simulink model "vier_Bit_Subtractor"  (R2024b)
settings: Solver=VariableStepAuto  StartTime=0.0  StopTime=10.0  RelTol=1e-3
libraries: simulink x3
settings Model: Creator=Steve Kinfack  LastModifiedBy=Steve Kinfack

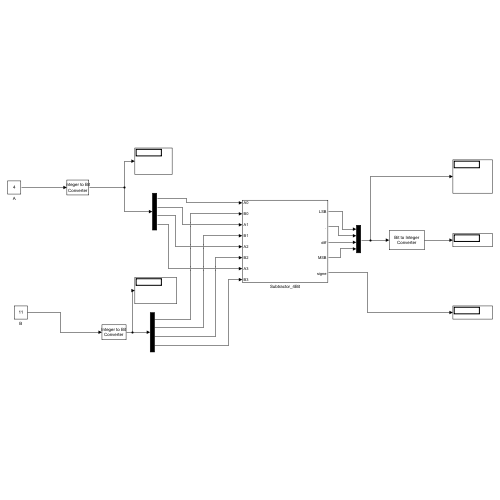
[thumbnail: Simulink's stored preview of the top-level diagram]
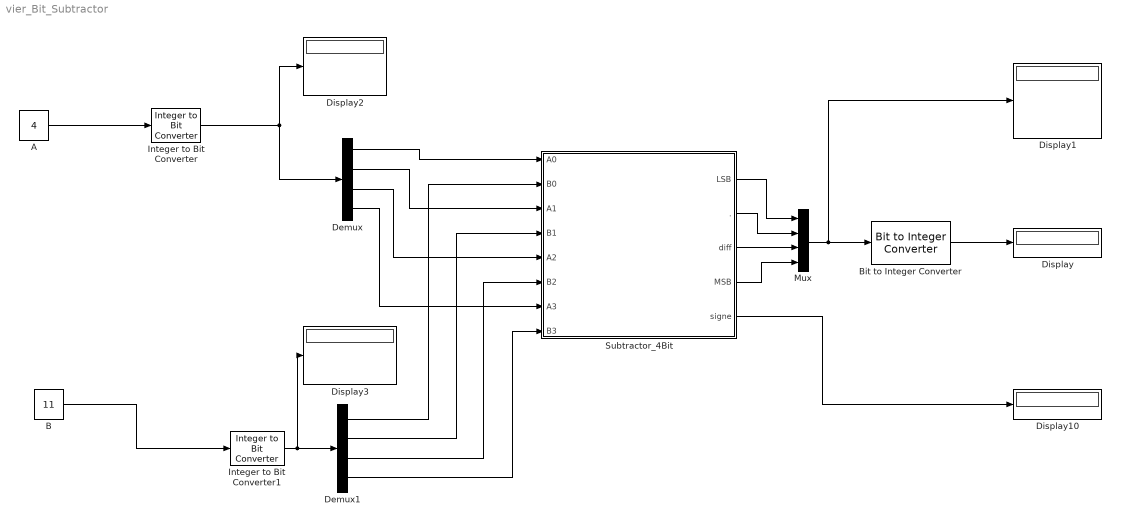
== system vier_Bit_Subtractor ==
  A : Constant  Value=4
  B : Constant  Value=11
  Bit to Integer Converter : simulink/Logic and Bit Operations/Bit to Integer Converter  nbits=4  bitOrder=LSB first  signedOutputValues=Unsigned  outDtype=Inherit via internal rule  outDtypeSigned=Inherit via internal rule
  Demux : Demux
  Demux1 : Demux
  Display{,1..3,10} (5 alike) : Display
  Integer to Bit Converter : simulink/Logic and Bit Operations/Integer to Bit Converter  nbits=4  signedInputValues=Unsigned  bitOrder=LSB first  outDtype=Inherit via internal rule
  Integer to Bit Converter1 : simulink/Logic and Bit Operations/Integer to Bit Converter  nbits=4  signedInputValues=Unsigned  bitOrder=LSB first  outDtype=Inherit via internal rule
  Mux : Mux
  Subtractor_4Bit : Subsystem
  wires:
  B/1 -> Integer to Bit Converter1/1
  Subtractor_4Bit/1(LSB) -> Mux/1
  Mux/1 -> Display1/1, Bit to Integer Converter/1
  Integer to Bit Converter/1 -> Demux/1, Display2/1
  Integer to Bit Converter1/1 -> Display3/1, Demux1/1
  Bit to Integer Converter/1 -> Display/1
  A/1 -> Integer to Bit Converter/1
  Subtractor_4Bit/2(.) -> Mux/2
  Subtractor_4Bit/3(diff) -> Mux/3
  Subtractor_4Bit/4(MSB) -> Mux/4
  Demux/1 -> Subtractor_4Bit/1(A0)
  Demux/2 -> Subtractor_4Bit/3(A1)
  Demux/3 -> Subtractor_4Bit/5(A2)
  Demux/4 -> Subtractor_4Bit/7(A3)
  Demux1/1 -> Subtractor_4Bit/2(B0)
  Demux1/2 -> Subtractor_4Bit/4(B1)
  Demux1/3 -> Subtractor_4Bit/6(B2)
  Demux1/4 -> Subtractor_4Bit/8(B3)
  Subtractor_4Bit/5(signe) -> Display10/1

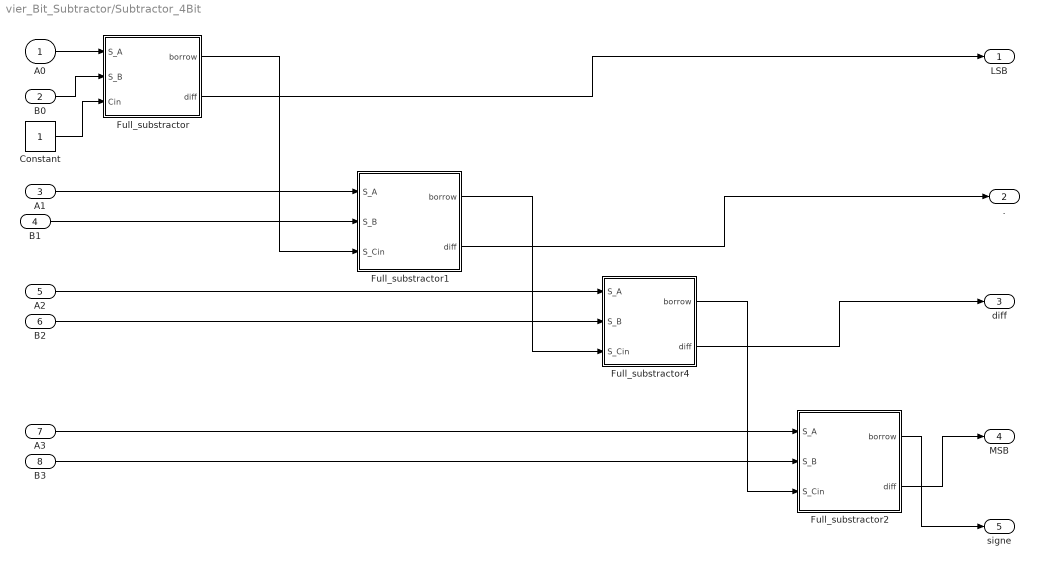
== system vier_Bit_Subtractor/Subtractor_4Bit ==
  A0 : Inport
  B0 : Inport  Port=2
  A1 : Inport  Port=3
  B1 : Inport  Port=4
  A2 : Inport  Port=5
  B2 : Inport  Port=6
  A3 : Inport  Port=7
  B3 : Inport  Port=8
  Constant : Constant
  Full_substractor : Subsystem
  Full_substractor1 : Subsystem
  Full_substractor2 : Subsystem
  Full_substractor4 : Subsystem
  LSB : Outport
  . : Outport  Port=2
  diff : Outport  Port=3
  MSB : Outport  Port=4
  signe : Outport  Port=5
  wires:
  A0/1 -> Full_substractor/1(S_A)
  B0/1 -> Full_substractor/2(S_B)
  A1/1 -> Full_substractor1/1(S_A)
  B1/1 -> Full_substractor1/2(S_B)
  A2/1 -> Full_substractor4/1(S_A)
  B2/1 -> Full_substractor4/2(S_B)
  A3/1 -> Full_substractor2/1(S_A)
  B3/1 -> Full_substractor2/2(S_B)
  Full_substractor/2(diff) -> LSB/1
  Constant/1 -> Full_substractor/3(Cin)
  Full_substractor/1(borrow) -> Full_substractor1/3(S_Cin)
  Full_substractor1/2(diff) -> ./1
  Full_substractor1/1(borrow) -> Full_substractor4/3(S_Cin)
  Full_substractor4/2(diff) -> diff/1
  Full_substractor4/1(borrow) -> Full_substractor2/3(S_Cin)
  Full_substractor2/2(diff) -> MSB/1
  Full_substractor2/1(borrow) -> signe/1

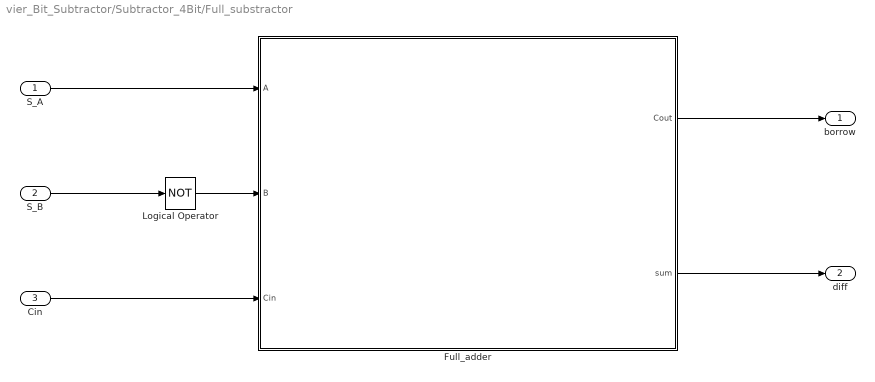
== system vier_Bit_Subtractor/Subtractor_4Bit/Full_substractor ==
  S_A : Inport
  S_B : Inport  Port=2
  Cin : Inport  Port=3
  Full_adder : Subsystem
  Logical Operator : Logic  Operator=NOT  AllPortsSameDT=off  OutDataTypeStr=boolean
  borrow : Outport
  diff : Outport  Port=2
  wires:
  S_B/1 -> Logical Operator/1
  Logical Operator/1 -> Full_adder/2(B)
  Cin/1 -> Full_adder/3(Cin)
  S_A/1 -> Full_adder/1(A)
  Full_adder/2(sum) -> diff/1
  Full_adder/1(Cout) -> borrow/1

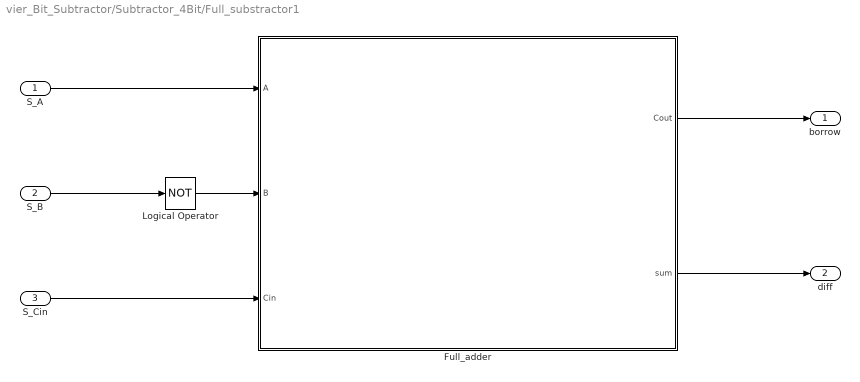
== system vier_Bit_Subtractor/Subtractor_4Bit/Full_substractor1 ==
  S_A : Inport
  S_B : Inport  Port=2
  S_Cin : Inport  Port=3
  Full_adder : Subsystem
  Logical Operator : Logic  Operator=NOT  AllPortsSameDT=off  OutDataTypeStr=boolean
  borrow : Outport
  diff : Outport  Port=2
  wires:
  S_B/1 -> Logical Operator/1
  Logical Operator/1 -> Full_adder/2(B)
  S_Cin/1 -> Full_adder/3(Cin)
  S_A/1 -> Full_adder/1(A)
  Full_adder/2(sum) -> diff/1
  Full_adder/1(Cout) -> borrow/1

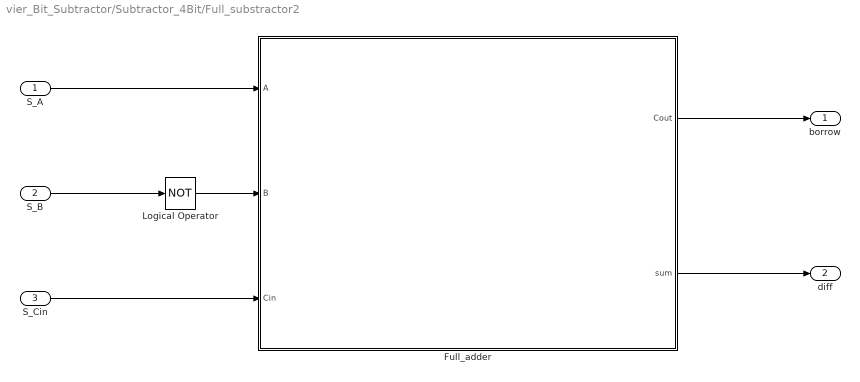
== system vier_Bit_Subtractor/Subtractor_4Bit/Full_substractor2 ==
  S_A : Inport
  S_B : Inport  Port=2
  S_Cin : Inport  Port=3
  Full_adder : Subsystem
  Logical Operator : Logic  Operator=NOT  AllPortsSameDT=off  OutDataTypeStr=boolean
  borrow : Outport
  diff : Outport  Port=2
  wires:
  S_B/1 -> Logical Operator/1
  Logical Operator/1 -> Full_adder/2(B)
  S_Cin/1 -> Full_adder/3(Cin)
  S_A/1 -> Full_adder/1(A)
  Full_adder/2(sum) -> diff/1
  Full_adder/1(Cout) -> borrow/1

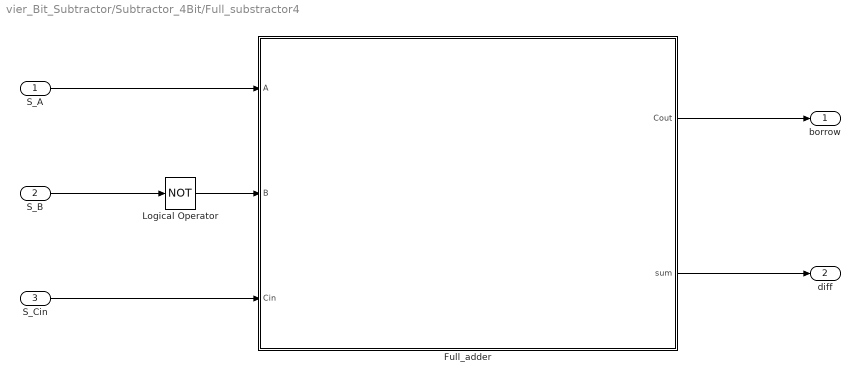
== system vier_Bit_Subtractor/Subtractor_4Bit/Full_substractor4 ==
  S_A : Inport
  S_B : Inport  Port=2
  S_Cin : Inport  Port=3
  Full_adder : Subsystem
  Logical Operator : Logic  Operator=NOT  AllPortsSameDT=off  OutDataTypeStr=boolean
  borrow : Outport
  diff : Outport  Port=2
  wires:
  S_B/1 -> Logical Operator/1
  Logical Operator/1 -> Full_adder/2(B)
  S_Cin/1 -> Full_adder/3(Cin)
  S_A/1 -> Full_adder/1(A)
  Full_adder/2(sum) -> diff/1
  Full_adder/1(Cout) -> borrow/1

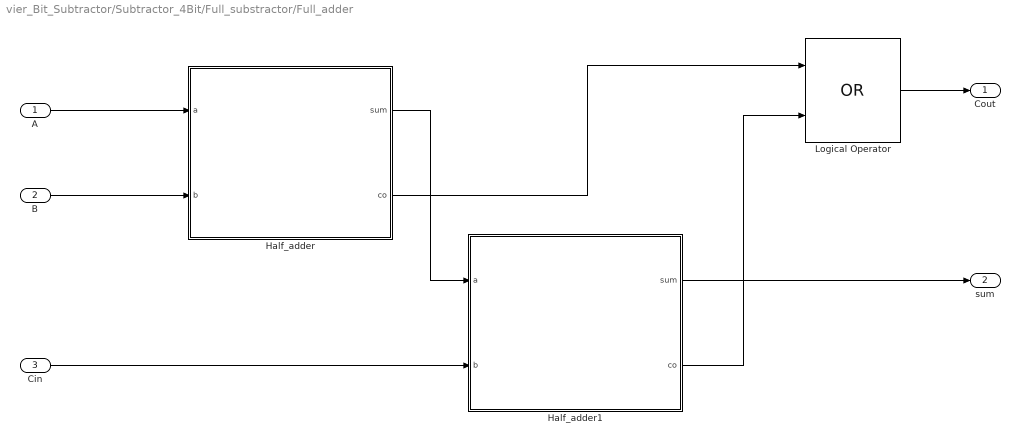
== system vier_Bit_Subtractor/Subtractor_4Bit/Full_substractor/Full_adder ==
  A : Inport
  B : Inport  Port=2
  Cin : Inport  Port=3
  Half_adder : Subsystem
  Half_adder1 : Subsystem
  Logical Operator : Logic  Operator=OR  AllPortsSameDT=off  OutDataTypeStr=boolean
  Cout : Outport
  sum : Outport  Port=2
  wires:
  A/1 -> Half_adder/1(a)
  B/1 -> Half_adder/2(b)
  Half_adder/1(sum) -> Half_adder1/1(a)
  Cin/1 -> Half_adder1/2(b)
  Half_adder/2(co) -> Logical Operator/1
  Half_adder1/2(co) -> Logical Operator/2
  Half_adder1/1(sum) -> sum/1
  Logical Operator/1 -> Cout/1

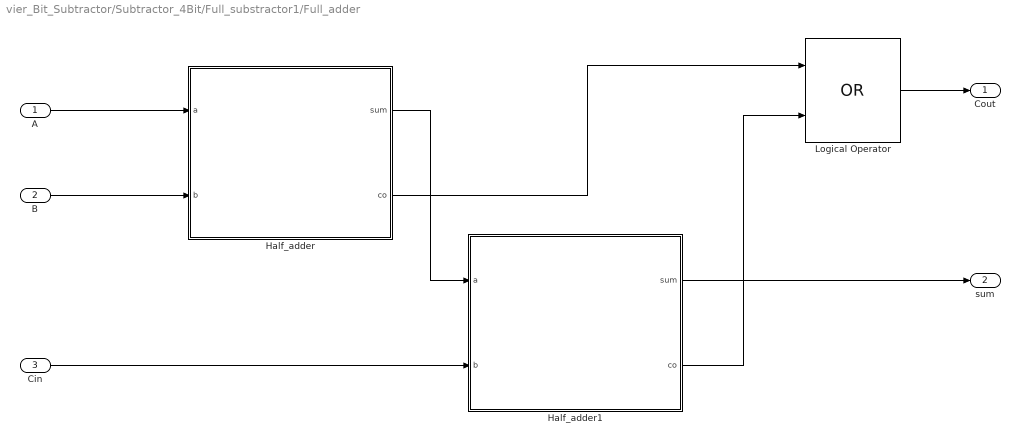
== system vier_Bit_Subtractor/Subtractor_4Bit/Full_substractor1/Full_adder ==
  A : Inport
  B : Inport  Port=2
  Cin : Inport  Port=3
  Half_adder : Subsystem
  Half_adder1 : Subsystem
  Logical Operator : Logic  Operator=OR  AllPortsSameDT=off  OutDataTypeStr=boolean
  Cout : Outport
  sum : Outport  Port=2
  wires:
  A/1 -> Half_adder/1(a)
  B/1 -> Half_adder/2(b)
  Half_adder/1(sum) -> Half_adder1/1(a)
  Cin/1 -> Half_adder1/2(b)
  Half_adder/2(co) -> Logical Operator/1
  Half_adder1/2(co) -> Logical Operator/2
  Half_adder1/1(sum) -> sum/1
  Logical Operator/1 -> Cout/1

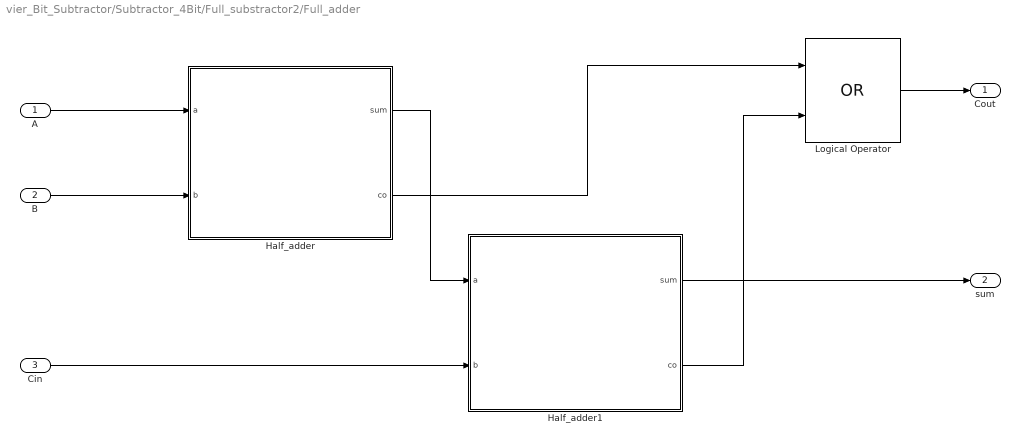
== system vier_Bit_Subtractor/Subtractor_4Bit/Full_substractor2/Full_adder ==
  A : Inport
  B : Inport  Port=2
  Cin : Inport  Port=3
  Half_adder : Subsystem
  Half_adder1 : Subsystem
  Logical Operator : Logic  Operator=OR  AllPortsSameDT=off  OutDataTypeStr=boolean
  Cout : Outport
  sum : Outport  Port=2
  wires:
  A/1 -> Half_adder/1(a)
  B/1 -> Half_adder/2(b)
  Half_adder/1(sum) -> Half_adder1/1(a)
  Cin/1 -> Half_adder1/2(b)
  Half_adder/2(co) -> Logical Operator/1
  Half_adder1/2(co) -> Logical Operator/2
  Half_adder1/1(sum) -> sum/1
  Logical Operator/1 -> Cout/1

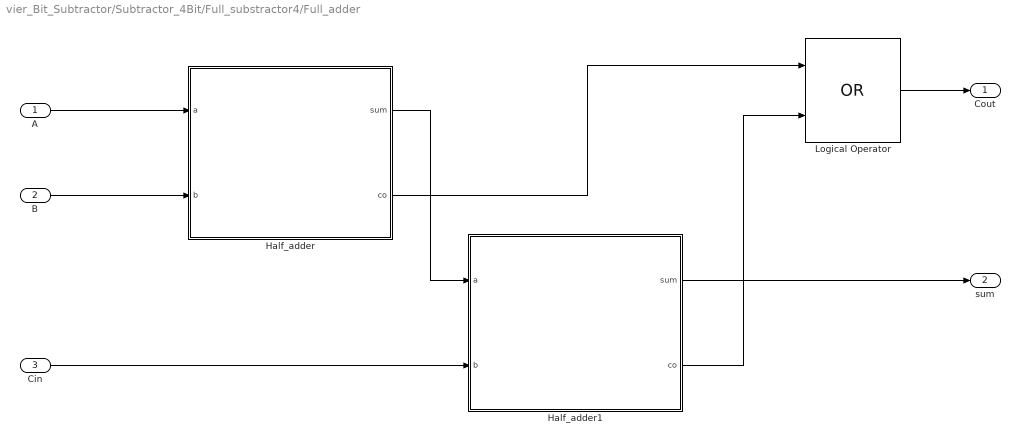
== system vier_Bit_Subtractor/Subtractor_4Bit/Full_substractor4/Full_adder ==
  A : Inport
  B : Inport  Port=2
  Cin : Inport  Port=3
  Half_adder : Subsystem
  Half_adder1 : Subsystem
  Logical Operator : Logic  Operator=OR  AllPortsSameDT=off  OutDataTypeStr=boolean
  Cout : Outport
  sum : Outport  Port=2
  wires:
  A/1 -> Half_adder/1(a)
  B/1 -> Half_adder/2(b)
  Half_adder/1(sum) -> Half_adder1/1(a)
  Cin/1 -> Half_adder1/2(b)
  Half_adder/2(co) -> Logical Operator/1
  Half_adder1/2(co) -> Logical Operator/2
  Half_adder1/1(sum) -> sum/1
  Logical Operator/1 -> Cout/1

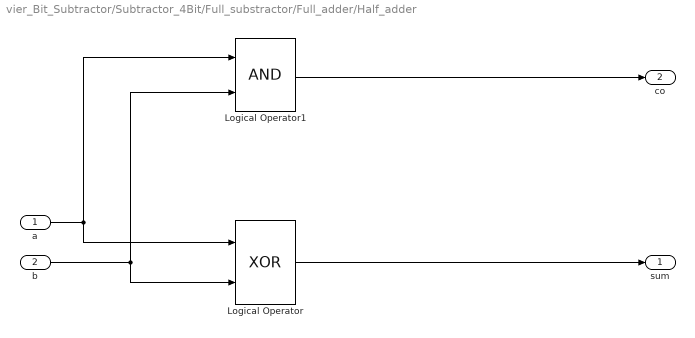
== system vier_Bit_Subtractor/Subtractor_4Bit/Full_substractor/Full_adder/Half_adder ==
  a : Inport
  b : Inport  Port=2
  Logical Operator : Logic  Operator=XOR  AllPortsSameDT=off  OutDataTypeStr=boolean
  Logical Operator1 : Logic  AllPortsSameDT=off  OutDataTypeStr=boolean
  sum : Outport
  co : Outport  Port=2
  wires:
  a/1 -> Logical Operator1/1, Logical Operator/1
  b/1 -> Logical Operator1/2, Logical Operator/2
  Logical Operator/1 -> sum/1
  Logical Operator1/1 -> co/1

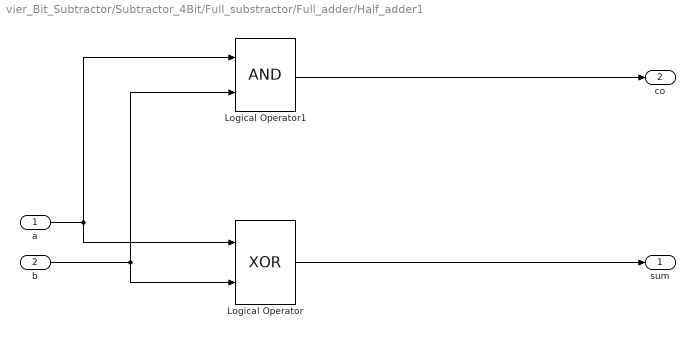
== system vier_Bit_Subtractor/Subtractor_4Bit/Full_substractor/Full_adder/Half_adder1 ==
  a : Inport
  b : Inport  Port=2
  Logical Operator : Logic  Operator=XOR  AllPortsSameDT=off  OutDataTypeStr=boolean
  Logical Operator1 : Logic  AllPortsSameDT=off  OutDataTypeStr=boolean
  sum : Outport
  co : Outport  Port=2
  wires:
  a/1 -> Logical Operator1/1, Logical Operator/1
  b/1 -> Logical Operator1/2, Logical Operator/2
  Logical Operator/1 -> sum/1
  Logical Operator1/1 -> co/1

== system vier_Bit_Subtractor/Subtractor_4Bit/Full_substractor1/Full_adder/Half_adder ==
  a : Inport
  b : Inport  Port=2
  Logical Operator : Logic  Operator=XOR  AllPortsSameDT=off  OutDataTypeStr=boolean
  Logical Operator1 : Logic  AllPortsSameDT=off  OutDataTypeStr=boolean
  sum : Outport
  co : Outport  Port=2
  wires:
  a/1 -> Logical Operator1/1, Logical Operator/1
  b/1 -> Logical Operator1/2, Logical Operator/2
  Logical Operator/1 -> sum/1
  Logical Operator1/1 -> co/1

== system vier_Bit_Subtractor/Subtractor_4Bit/Full_substractor1/Full_adder/Half_adder1 ==
  a : Inport
  b : Inport  Port=2
  Logical Operator : Logic  Operator=XOR  AllPortsSameDT=off  OutDataTypeStr=boolean
  Logical Operator1 : Logic  AllPortsSameDT=off  OutDataTypeStr=boolean
  sum : Outport
  co : Outport  Port=2
  wires:
  a/1 -> Logical Operator1/1, Logical Operator/1
  b/1 -> Logical Operator1/2, Logical Operator/2
  Logical Operator/1 -> sum/1
  Logical Operator1/1 -> co/1

== system vier_Bit_Subtractor/Subtractor_4Bit/Full_substractor2/Full_adder/Half_adder ==
  a : Inport
  b : Inport  Port=2
  Logical Operator : Logic  Operator=XOR  AllPortsSameDT=off  OutDataTypeStr=boolean
  Logical Operator1 : Logic  AllPortsSameDT=off  OutDataTypeStr=boolean
  sum : Outport
  co : Outport  Port=2
  wires:
  a/1 -> Logical Operator1/1, Logical Operator/1
  b/1 -> Logical Operator1/2, Logical Operator/2
  Logical Operator/1 -> sum/1
  Logical Operator1/1 -> co/1

== system vier_Bit_Subtractor/Subtractor_4Bit/Full_substractor2/Full_adder/Half_adder1 ==
  a : Inport
  b : Inport  Port=2
  Logical Operator : Logic  Operator=XOR  AllPortsSameDT=off  OutDataTypeStr=boolean
  Logical Operator1 : Logic  AllPortsSameDT=off  OutDataTypeStr=boolean
  sum : Outport
  co : Outport  Port=2
  wires:
  a/1 -> Logical Operator1/1, Logical Operator/1
  b/1 -> Logical Operator1/2, Logical Operator/2
  Logical Operator/1 -> sum/1
  Logical Operator1/1 -> co/1

== system vier_Bit_Subtractor/Subtractor_4Bit/Full_substractor4/Full_adder/Half_adder ==
  a : Inport
  b : Inport  Port=2
  Logical Operator : Logic  Operator=XOR  AllPortsSameDT=off  OutDataTypeStr=boolean
  Logical Operator1 : Logic  AllPortsSameDT=off  OutDataTypeStr=boolean
  sum : Outport
  co : Outport  Port=2
  wires:
  a/1 -> Logical Operator1/1, Logical Operator/1
  b/1 -> Logical Operator1/2, Logical Operator/2
  Logical Operator/1 -> sum/1
  Logical Operator1/1 -> co/1

== system vier_Bit_Subtractor/Subtractor_4Bit/Full_substractor4/Full_adder/Half_adder1 ==
  a : Inport
  b : Inport  Port=2
  Logical Operator : Logic  Operator=XOR  AllPortsSameDT=off  OutDataTypeStr=boolean
  Logical Operator1 : Logic  AllPortsSameDT=off  OutDataTypeStr=boolean
  sum : Outport
  co : Outport  Port=2
  wires:
  a/1 -> Logical Operator1/1, Logical Operator/1
  b/1 -> Logical Operator1/2, Logical Operator/2
  Logical Operator/1 -> sum/1
  Logical Operator1/1 -> co/1
